simulink model "model"  (Simulink 7.3)
settings: Solver=ode45  StartTime=0.0  StopTime=2  RelTol=1e-3
values from neighbouring files (symbols this model uses):
  C_bp = 0.358    [init.m]
  C_bv = 10.71    [init.m]
  C_ep = 0.668    [init.m]
  C_ev = 20    [init.m]
  C_hp = 0.119    [init.m]
  C_hv = 3.57    [init.m]
  C_la = 19.23    [init.m]
  C_mp = 0.525    [init.m]
  C_mv = 15.71    [init.m]
  C_pa = 0.76    [init.m]
  C_pp = 5.8    [init.m]
  C_pv = 25.37    [init.m]
  C_ra = 31.25    [init.m]
  C_sa = 0.28    [init.m]
  C_sp = 2.05    [init.m]
  C_sv = 61.11    [init.m]
  D_E_max_lv = 2    [init.m]
  D_E_max_rv = 2    [init.m]
  D_R_ep = 2    [init.m]
  D_R_mp = 2    [init.m]
  D_R_sp = 2    [init.m]
  D_T_s = 2    [init.m]
  D_T_v = 0.02    [init.m]
  D_u_ev = 5    [init.m]
  D_u_mv = 5    [init.m]
  D_u_sv = 5    [init.m]
  D_v = 6    [init.m]
  E_max_lv_0 = 2.392    [init.m]
  E_max_rv_0 = 1.412    [init.m]
  f_ab_0 = 1    [init.m]
  f_abmax = 47.78    [init.m]
  f_abmin = 0    [init.m]
  f_ac_max = 17.07    [init.m]
  f_ac_min = 0    [init.m]
  f_ac_n = 3.6    [init.m]
  f_es_0 = 16.11    [init.m]
  f_es_inf = 2.1    [init.m]
  f_es_max = 60    [init.m]
  f_es_min = 0    [init.m]
  f_ev_0 = 3.2    [init.m]
  f_ev_inf = 6.3    [init.m]
  fi_sh = 0    [init.m]
  fi_sp = 0    [init.m]
  fi_v = -0.68    [init.m]
  G_ap = 23.29    [init.m]
  G_E_max_lv = 0.475    [init.m]
  G_E_max_rv = 0.282    [init.m]
  G_R_ep = 1.94    [init.m]
  G_R_mp = 2.47    [init.m]
  G_R_sp = 0.695    [init.m]
  G_T_s = -0.13    [init.m]
  G_T_v = 0.09    [init.m]
  G_u_ev = -74.21    [init.m]
  G_u_mv = -58.29    [init.m]
  G_u_sv = -265.4    [init.m]
  G_v = 0.125    [init.m]
  k_a_b = 11.76    [init.m]
  k_ac = 29.27    [init.m]
  k_e_lv = 0.014    [init.m]
  k_e_rv = 0.011    [init.m]
  k_es = 0.0675    [init.m]
  k_ev = 7.06    [init.m]
  k_r_lv = 0.000375    [init.m]
  k_r_rv = 0.0014    [init.m]
  k_sys = 0.075    [init.m]
  L_pa = 0.00018    [init.m]
  p_as_o2 = 30    [init.m]
  p_as_o2_n = 45    [init.m]
  p_n = 92    [init.m]
  P_o_lv = 1.5    [init.m]
  P_o_rv = 1.5    [init.m]
  R_bp = 6.57    [init.m]
  R_bv = 0.075    [init.m]
  R_ep_0 = 1.655    [init.m]
  R_ev = 0.04    [init.m]
  R_hp = 19.71    [init.m]
  R_hv = 0.224    [init.m]
  R_la = 0.0025    [init.m]
  R_mp_0 = 2.106    [init.m]
  R_mv = 0.05    [init.m]
  R_pa = 0.023    [init.m]
  R_pp = 0.0894    [init.m]
  R_pv = 0.0056    [init.m]
  R_ra = 0.0025    [init.m]
  R_sa = 0.06    [init.m]
  R_sp_0 = 2.49    [init.m]
  R_sv = 0.038    [init.m]
  T_0 = 0.58    [init.m]
  T_sys_0 = 0.5    [init.m]
  tau_c = 2    [init.m]
  tau_E_max_rv = 8    [init.m]
  tau_p = 2    [init.m]
  tau_pb = 2.076    [init.m]
  tau_R_ep = 6    [init.m]
  tau_R_mp = 6    [init.m]
  tau_R_sp = 6    [init.m]
  tau_T_s = 2    [init.m]
  tau_T_v = 1.5    [init.m]
  tau_u_ev = 20    [init.m]
  tau_u_mv = 20    [init.m]
  tau_u_sv = 20    [init.m]
  tau_v = 3    [init.m]
  tau_zb = 6.37    [init.m]
  V_tn = 0.583    [init.m]
  V_tot = 5300    [init.m]
  V_u_bp = 72.13    [init.m]
  V_u_bv = 294.64    [init.m]
  V_u_ep = 134.64    [init.m]
  V_u_ev_0 = 640.73    [init.m]
  V_u_hp = 24    [init.m]
  V_u_hv = 98.21    [init.m]
  V_u_la = 25    [init.m]
  V_u_lv = 16.77    [init.m]
  V_u_mp = 105.8    [init.m]
  V_u_mv_0 = 503.26    [init.m]
  V_u_pa = 0    [init.m]
  V_u_pp = 123    [init.m]
  V_u_pv = 120    [init.m]
  V_u_ra = 25    [init.m]
  V_u_rv = 40.8    [init.m]
  ... (+11 more)
(part 2 of 2)

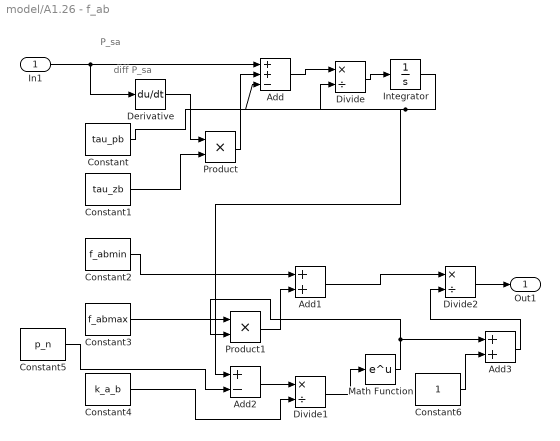
== system model/A1.26 - f_ab ==
  note: P_sa
  note: diff P_sa
  In1 : Inport  OutDataType=fixdt(1, 16)  OutScaling=2^0
  Add : Sum  Inputs=++-  OutDataType=fixdt(1, 16)  OutScaling=2^-10
  Add1 : Sum  OutDataType=fixdt(1, 16)  OutScaling=2^-10
  Add2 : Sum  Inputs=+-  OutDataType=fixdt(1, 16)  OutScaling=2^-10
  Add3 : Sum  OutDataType=fixdt(1, 16)  OutScaling=2^-10
  Constant : Constant  Value=tau_pb  OutDataType=fixdt(1, 16)  OutScaling=2^0
  Constant1 : Constant  Value=tau_zb  OutDataType=fixdt(1, 16)  OutScaling=2^0
  Constant2 : Constant  Value=f_abmin  OutDataType=fixdt(1, 16)  OutScaling=2^0
  Constant3 : Constant  Value=f_abmax  OutDataType=fixdt(1, 16)  OutScaling=2^0
  Constant4 : Constant  Value=k_a_b  OutDataType=fixdt(1, 16)  OutScaling=2^0
  Constant5 : Constant  Value=p_n  OutDataType=fixdt(1, 16)  OutScaling=2^0
  Constant6 : Constant  OutDataType=fixdt(1, 16)  OutScaling=2^0
  Derivative : Derivative
  Divide : Product  Inputs=*/  OutDataType=fixdt(1, 16)  OutScaling=2^-10
  Divide1 : Product  Inputs=*/  OutDataType=fixdt(1, 16)  OutScaling=2^-10
  Divide2 : Product  Inputs=*/  OutDataType=fixdt(1, 16)  OutScaling=2^-10
  Integrator : Integrator  InitialCondition=1
  Math Function : Math  OutDataType=fixdt(1, 16)  OutScaling=2^0  SaturateOnIntegerOverflow=on
  Product : Product  OutDataType=fixdt(1, 16)  OutScaling=2^0  RndMeth=Zero
  Product1 : Product  OutDataType=fixdt(1, 16)  OutScaling=2^0  RndMeth=Zero
  Out1 : Outport  OutDataType=fixdt(1, 16)  OutScaling=2^0
  wires:
  Constant1/1 -> Product/2
  Product/1 -> Add/2
  Integrator/1 -> Add/3, Add2/1
  Add/1 -> Divide/1
  Constant/1 -> Divide/2
  Divide/1 -> Integrator/1
  Constant2/1 -> Add1/1
  Constant3/1 -> Product1/1
  Add2/1 -> Divide1/1
  Constant5/1 -> Add2/2
  Constant4/1 -> Divide1/2
  Divide1/1 -> Math Function/1
  Math Function/1 -> Product1/2, Add3/1
  Product1/1 -> Add1/2
  Constant6/1 -> Add3/2
  Add3/1 -> Divide2/2
  Add1/1 -> Divide2/1
  Divide2/1 -> Out1/1
  Derivative/1 -> Product/1
  In1/1 -> Add/1, Derivative/1

== system model/A1.27 - f_ac ==
  Add : Sum  OutDataType=fixdt(1, 16)  OutScaling=2^-10
  Add1 : Sum  Inputs=+-  OutDataType=fixdt(1, 16)  OutScaling=2^-10
  Add2 : Sum  OutDataType=fixdt(1, 16)  OutScaling=2^-10
  Add3 : Sum  Inputs=+-  OutDataType=fixdt(1, 16)  OutScaling=2^-10
  Constant : Constant  Value=f_ac_max  OutDataType=fixdt(1, 16)  OutScaling=2^0
  Constant1 : Constant  Value=p_as_o2  OutDataType=fixdt(1, 16)  OutScaling=2^0
  Constant2 : Constant  Value=p_as_o2_n  OutDataType=fixdt(1, 16)  OutScaling=2^0
  Constant3 : Constant  Value=k_ac  OutDataType=fixdt(1, 16)  OutScaling=2^0
  Constant4 : Constant  Value=f_ac_min  OutDataType=fixdt(1, 16)  OutScaling=2^0
  Constant5 : Constant  OutDataType=fixdt(1, 16)  OutScaling=2^0
  Constant6 : Constant  Value=tau_c  OutDataType=fixdt(1, 16)  OutScaling=2^0
  Divide : Product  Inputs=*/  OutDataType=fixdt(1, 16)  OutScaling=2^-10
  Divide1 : Product  Inputs=*/  OutDataType=fixdt(1, 16)  OutScaling=2^-10
  Divide2 : Product  Inputs=*/  OutDataType=fixdt(1, 16)  OutScaling=2^-10
  Integrator : Integrator  InitialCondition=1
  Math Function : Math  OutDataType=fixdt(1, 16)  OutScaling=2^0  SaturateOnIntegerOverflow=on
  Product : Product  OutDataType=fixdt(1, 16)  OutScaling=2^0  RndMeth=Zero
  Out1 : Outport  OutDataType=fixdt(1, 16)  OutScaling=2^0
  wires:
  Constant/1 -> Add/1
  Constant1/1 -> Add1/1
  Constant2/1 -> Add1/2
  Add1/1 -> Divide/1
  Constant3/1 -> Divide/2
  Divide/1 -> Math Function/1
  Math Function/1 -> Product/2, Add2/1
  Constant4/1 -> Product/1
  Product/1 -> Add/2
  Constant5/1 -> Add2/2
  Add2/1 -> Divide1/2
  Add/1 -> Divide1/1
  Integrator/1 -> Add3/2, Out1/1
  Divide1/1 -> Add3/1
  Add3/1 -> Divide2/1
  Constant6/1 -> Divide2/2
  Divide2/1 -> Integrator/1

== system model/A1.28 - f_ap ==
  note: V_t
  In1 : Inport  OutDataType=fixdt(1, 16)  OutScaling=2^0
  Add : Sum  Inputs=-+  OutDataType=fixdt(1, 16)  OutScaling=2^-10
  Constant : Constant  Value=G_ap  OutDataType=fixdt(1, 16)  OutScaling=2^0
  Constant1 : Constant  Value=tau_p  OutDataType=fixdt(1, 16)  OutScaling=2^0
  Divide : Product  Inputs=*/  OutDataType=fixdt(1, 16)  OutScaling=2^-10
  Integrator : Integrator  InitialCondition=1
  Product : Product  OutDataType=fixdt(1, 16)  OutScaling=2^0  RndMeth=Zero
  Out1 : Outport  OutDataType=fixdt(1, 16)  OutScaling=2^0
  wires:
  Constant/1 -> Product/1
  Product/1 -> Add/2
  Integrator/1 -> Add/1, Out1/1
  Add/1 -> Divide/1
  Constant1/1 -> Divide/2
  Divide/1 -> Integrator/1
  In1/1 -> Product/2

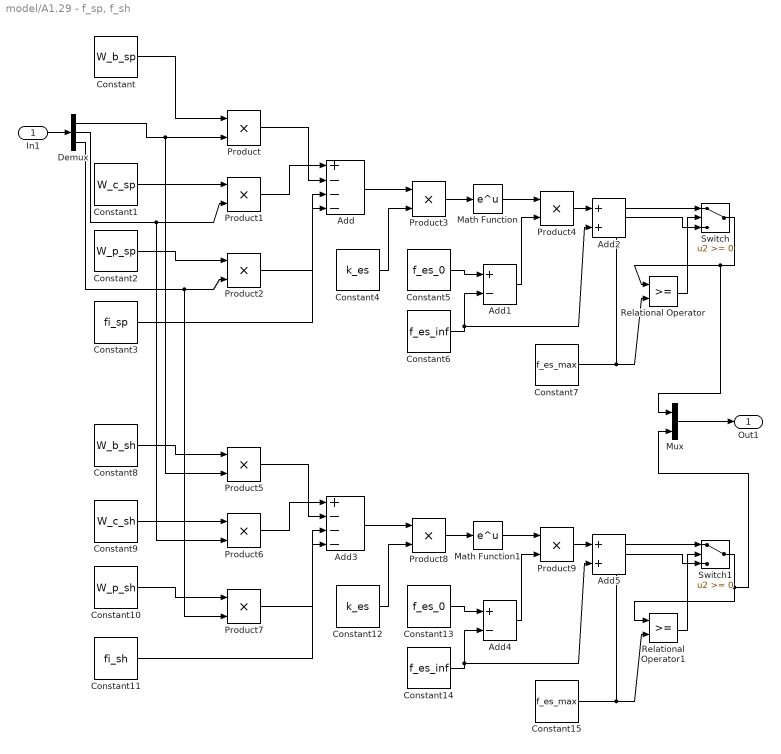
== system model/A1.29 - f_sp, f_sh ==
  In1 : Inport  OutDataType=fixdt(1, 16)  OutScaling=2^0
  Add : Sum  Inputs=+---  OutDataType=fixdt(1, 16)  OutScaling=2^-10
  Add1 : Sum  Inputs=+-  OutDataType=fixdt(1, 16)  OutScaling=2^-10
  Add2 : Sum  OutDataType=fixdt(1, 16)  OutScaling=2^-10
  Add3 : Sum  Inputs=+---  OutDataType=fixdt(1, 16)  OutScaling=2^-10
  Add4 : Sum  Inputs=+-  OutDataType=fixdt(1, 16)  OutScaling=2^-10
  Add5 : Sum  OutDataType=fixdt(1, 16)  OutScaling=2^-10
  Constant : Constant  Value=W_b_sp  OutDataType=fixdt(1, 16)  OutScaling=2^0
  Constant1 : Constant  Value=W_c_sp  OutDataType=fixdt(1, 16)  OutScaling=2^0
  Constant10 : Constant  Value=W_p_sh  OutDataType=fixdt(1, 16)  OutScaling=2^0
  Constant11 : Constant  Value=fi_sh  OutDataType=fixdt(1, 16)  OutScaling=2^0
  Constant12 : Constant  Value=k_es  OutDataType=fixdt(1, 16)  OutScaling=2^0
  Constant13 : Constant  Value=f_es_0  OutDataType=fixdt(1, 16)  OutScaling=2^0
  Constant14 : Constant  Value=f_es_inf  OutDataType=fixdt(1, 16)  OutScaling=2^0
  Constant15 : Constant  Value=f_es_max  OutDataType=fixdt(1, 16)  OutScaling=2^0
  Constant2 : Constant  Value=W_p_sp  OutDataType=fixdt(1, 16)  OutScaling=2^0
  Constant3 : Constant  Value=fi_sp  OutDataType=fixdt(1, 16)  OutScaling=2^0
  Constant4 : Constant  Value=k_es  OutDataType=fixdt(1, 16)  OutScaling=2^0
  Constant5 : Constant  Value=f_es_0  OutDataType=fixdt(1, 16)  OutScaling=2^0
  Constant6 : Constant  Value=f_es_inf  OutDataType=fixdt(1, 16)  OutScaling=2^0
  Constant7 : Constant  Value=f_es_max  OutDataType=fixdt(1, 16)  OutScaling=2^0
  Constant8 : Constant  Value=W_b_sh  OutDataType=fixdt(1, 16)  OutScaling=2^0
  Constant9 : Constant  Value=W_c_sh  OutDataType=fixdt(1, 16)  OutScaling=2^0
  Demux : Demux  Outputs=3
  Math Function : Math  OutDataType=fixdt(1, 16)  OutScaling=2^0  SaturateOnIntegerOverflow=on
  Math Function1 : Math  OutDataType=fixdt(1, 16)  OutScaling=2^0  SaturateOnIntegerOverflow=on
  Mux : Mux  Inputs=2
  Product{,1..9} (10 alike) : Product  OutDataType=fixdt(1, 16)  OutScaling=2^0  RndMeth=Zero
  Relational Operator : RelationalOperator  LogicOutDataTypeMode=boolean  LogicDataType=fixdt(0, 8)  OutDataTypeStr=boolean
  Relational Operator1 : RelationalOperator  LogicOutDataTypeMode=boolean  LogicDataType=fixdt(0, 8)  OutDataTypeStr=boolean
  Switch : Switch  OutDataType=fixdt(1, 16)  OutScaling=2^0
  Switch1 : Switch  OutDataType=fixdt(1, 16)  OutScaling=2^0
  Out1 : Outport  OutDataType=fixdt(1, 16)  OutScaling=2^0
  wires:
  In1/1 -> Demux/1
  Demux/1 -> Product/2, Product5/2
  Constant1/1 -> Product1/1
  Demux/2 -> Product1/2, Product6/2
  Constant2/1 -> Product2/1
  Demux/3 -> Product2/2, Product7/2
  Constant/1 -> Product/1
  Product1/1 -> Add/1
  Product/1 -> Add/2
  Product2/1 -> Add/3
  Constant3/1 -> Add/4
  Add/1 -> Product3/1
  Constant4/1 -> Product3/2
  Product3/1 -> Math Function/1
  Math Function/1 -> Product4/1
  Constant5/1 -> Add1/1
  Constant6/1 -> Add1/2, Add2/2
  Add1/1 -> Product4/2
  Product4/1 -> Add2/1
  Switch/1 -> Relational Operator/1, Mux/1
  Constant7/1 -> Relational Operator/2, Switch/1
  Relational Operator/1 -> Switch/2
  Add2/1 -> Switch/3
  Constant9/1 -> Product6/1
  Constant10/1 -> Product7/1
  Constant8/1 -> Product5/1
  Product6/1 -> Add3/1
  Product5/1 -> Add3/2
  Product7/1 -> Add3/3
  Constant11/1 -> Add3/4
  Add3/1 -> Product8/1
  Constant12/1 -> Product8/2
  Product8/1 -> Math Function1/1
  Math Function1/1 -> Product9/1
  Constant13/1 -> Add4/1
  Constant14/1 -> Add4/2, Add5/2
  Add4/1 -> Product9/2
  Product9/1 -> Add5/1
  Switch1/1 -> Relational Operator1/1, Mux/2
  Constant15/1 -> Relational Operator1/2, Switch1/1
  Relational Operator1/1 -> Switch1/2
  Add5/1 -> Switch1/3
  Mux/1 -> Out1/1

== system model/A1.3 - P_pp ==
  note: P pv
  note: F pa
  In1 : Inport  OutDataType=fixdt(1, 16)  OutScaling=2^0
  Constant : Constant  Value=R_pp  OutDataType=fixdt(1, 16)  OutScaling=2^0
  Constant1 : Constant  Value=C_pp  OutDataType=fixdt(1, 16)  OutScaling=2^0
  Demux : Demux  Outputs=2
  Divide : Product  Inputs=*/  OutDataType=fixdt(1, 16)  OutScaling=2^-10
  Divide1 : Product  Inputs=*/  OutDataType=fixdt(1, 16)  OutScaling=2^-10
  Integrator : Integrator  InitialCondition=1
  Subtract : Sum  Inputs=+-  OutDataType=fixdt(1, 16)  OutScaling=2^-10
  Subtract1 : Sum  Inputs=+-  OutDataType=fixdt(1, 16)  OutScaling=2^-10
  Out1 : Outport  OutDataType=fixdt(1, 16)  OutScaling=2^0
  wires:
  In1/1 -> Demux/1
  Subtract/1 -> Divide/1
  Constant/1 -> Divide/2
  Constant1/1 -> Divide1/2
  Subtract1/1 -> Divide1/1
  Divide1/1 -> Integrator/1
  Integrator/1 -> Out1/1, Subtract/1
  Divide/1 -> Subtract1/2
  Demux/1 -> Subtract/2
  Demux/2 -> Subtract1/1

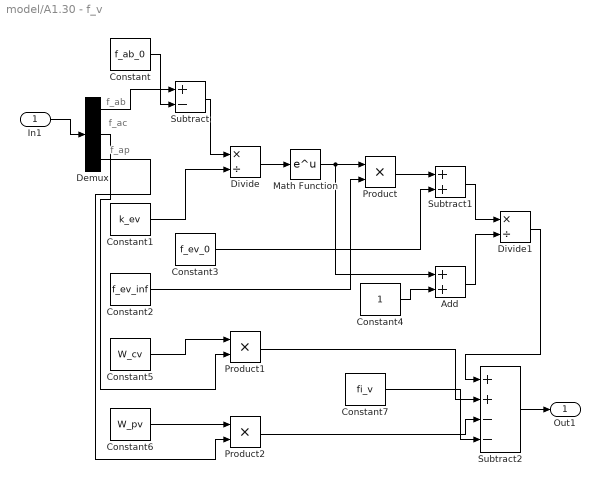
== system model/A1.30 - f_v  ==
  note: f_ab
  note: f_ac
  note: f_ap
  In1 : Inport  OutDataType=fixdt(1, 16)  OutScaling=2^0
  Add : Sum  OutDataType=fixdt(1, 16)  OutScaling=2^-10
  Constant : Constant  Value=f_ab_0  OutDataType=fixdt(1, 16)  OutScaling=2^0
  Constant1 : Constant  Value=k_ev  OutDataType=fixdt(1, 16)  OutScaling=2^0
  Constant2 : Constant  Value=f_ev_inf  OutDataType=fixdt(1, 16)  OutScaling=2^0
  Constant3 : Constant  Value=f_ev_0  OutDataType=fixdt(1, 16)  OutScaling=2^0
  Constant4 : Constant  OutDataType=fixdt(1, 16)  OutScaling=2^0
  Constant5 : Constant  Value=W_cv  OutDataType=fixdt(1, 16)  OutScaling=2^0
  Constant6 : Constant  Value=W_pv  OutDataType=fixdt(1, 16)  OutScaling=2^0
  Constant7 : Constant  Value=fi_v  OutDataType=fixdt(1, 16)  OutScaling=2^0
  Demux : Demux  Outputs=3
  Divide : Product  Inputs=*/  OutDataType=fixdt(1, 16)  OutScaling=2^-10
  Divide1 : Product  Inputs=*/  OutDataType=fixdt(1, 16)  OutScaling=2^-10
  Math Function : Math  OutDataType=fixdt(1, 16)  OutScaling=2^0  SaturateOnIntegerOverflow=on
  Product : Product  OutDataType=fixdt(1, 16)  OutScaling=2^0  RndMeth=Zero
  Product1 : Product  OutDataType=fixdt(1, 16)  OutScaling=2^0  RndMeth=Zero
  Product2 : Product  OutDataType=fixdt(1, 16)  OutScaling=2^0  RndMeth=Zero
  Subtract : Sum  Inputs=+-  OutDataType=fixdt(1, 16)  OutScaling=2^-10
  Subtract1 : Sum  OutDataType=fixdt(1, 16)  OutScaling=2^-10
  Subtract2 : Sum  Inputs=++--  OutDataType=fixdt(1, 16)  OutScaling=2^-10
  Out1 : Outport  OutDataType=fixdt(1, 16)  OutScaling=2^0
  wires:
  In1/1 -> Demux/1
  Demux/1 -> Subtract/1
  Constant/1 -> Subtract/2
  Subtract/1 -> Divide/1
  Constant1/1 -> Divide/2
  Divide/1 -> Math Function/1
  Math Function/1 -> Product/1, Add/1
  Constant2/1 -> Product/2
  Product/1 -> Subtract1/1
  Constant3/1 -> Subtract1/2
  Constant4/1 -> Add/2
  Add/1 -> Divide1/2
  Subtract1/1 -> Divide1/1
  Constant5/1 -> Product1/1
  Demux/2 -> Product1/2
  Constant6/1 -> Product2/1
  Demux/3 -> Product2/2
  Divide1/1 -> Subtract2/1
  Product1/1 -> Subtract2/2
  Product2/1 -> Subtract2/3
  Constant7/1 -> Subtract2/4
  Subtract2/1 -> Out1/1

== system model/A1.4 - P_pv ==
  note: P pp
  note: P la
  In1 : Inport  OutDataType=fixdt(1, 16)  OutScaling=2^0
  Constant : Constant  Value=R_pp  OutDataType=fixdt(1, 16)  OutScaling=2^0
  Constant1 : Constant  Value=R_pv  OutDataType=fixdt(1, 16)  OutScaling=2^0
  Constant2 : Constant  Value=C_pv  OutDataType=fixdt(1, 16)  OutScaling=2^0
  Demux : Demux  Outputs=2
  Divide : Product  Inputs=*/  OutDataType=fixdt(1, 16)  OutScaling=2^-10
  Divide1 : Product  Inputs=*/  OutDataType=fixdt(1, 16)  OutScaling=2^-10
  Divide2 : Product  Inputs=*/  OutDataType=fixdt(1, 16)  OutScaling=2^-10
  Integrator : Integrator  InitialCondition=1
  Subtract : Sum  Inputs=+-  OutDataType=fixdt(1, 16)  OutScaling=2^-10
  Subtract1 : Sum  Inputs=+-  OutDataType=fixdt(1, 16)  OutScaling=2^-10
  Subtract2 : Sum  Inputs=+-  OutDataType=fixdt(1, 16)  OutScaling=2^-10
  Out1 : Outport  OutDataType=fixdt(1, 16)  OutScaling=2^0
  wires:
  In1/1 -> Demux/1
  Demux/1 -> Subtract/1
  Demux/2 -> Subtract1/2
  Integrator/1 -> Out1/1, Subtract/2, Subtract1/1
  Subtract/1 -> Divide/1
  Constant/1 -> Divide/2
  Subtract1/1 -> Divide1/1
  Constant1/1 -> Divide1/2
  Divide/1 -> Subtract2/1
  Divide1/1 -> Subtract2/2
  Subtract2/1 -> Divide2/1
  Constant2/1 -> Divide2/2
  Divide2/1 -> Integrator/1

== system model/A1.5 - P_sa ==
  note: F o,l
  note: F sa
  In1 : Inport  OutDataType=fixdt(1, 16)  OutScaling=2^0
  Constant : Constant  Value=C_sa  OutDataType=fixdt(1, 16)  OutScaling=2^0
  Demux : Demux  Outputs=2
  Divide : Product  Inputs=*/  OutDataType=fixdt(1, 16)  OutScaling=2^-10
  Integrator : Integrator  InitialCondition=1
  Subtract : Sum  Inputs=+-  OutDataType=fixdt(1, 16)  OutScaling=2^-10
  Out1 : Outport  OutDataType=fixdt(1, 16)  OutScaling=2^0
  wires:
  In1/1 -> Demux/1
  Demux/1 -> Subtract/1
  Demux/2 -> Subtract/2
  Subtract/1 -> Divide/1
  Constant/1 -> Divide/2
  Divide/1 -> Integrator/1
  Integrator/1 -> Out1/1

== system model/A1.6 - F_sa ==
  note: P sa
  note: P sp
  note: F sa
  In1 : Inport  OutDataType=fixdt(1, 16)  OutScaling=2^0
  Constant : Constant  Value=R_sa  OutDataType=fixdt(1, 16)  OutScaling=2^0
  Demux : Demux  Outputs=2
  Integrator : Integrator  InitialCondition=1
  Product : Product  OutDataType=fixdt(1, 16)  OutScaling=2^0  RndMeth=Zero
  Subtract : Sum  Inputs=+-  OutDataType=fixdt(1, 16)  OutScaling=2^-10
  Subtract1 : Sum  Inputs=+-  OutDataType=fixdt(1, 16)  OutScaling=2^-10
  Out1 : Outport  OutDataType=fixdt(1, 16)  OutScaling=2^0
  wires:
  In1/1 -> Demux/1
  Demux/1 -> Subtract/1
  Demux/2 -> Subtract/2
  Constant/1 -> Product/1
  Subtract/1 -> Subtract1/1
  Product/1 -> Subtract1/2
  Subtract1/1 -> Integrator/1
  Integrator/1 -> Out1/1, Product/2

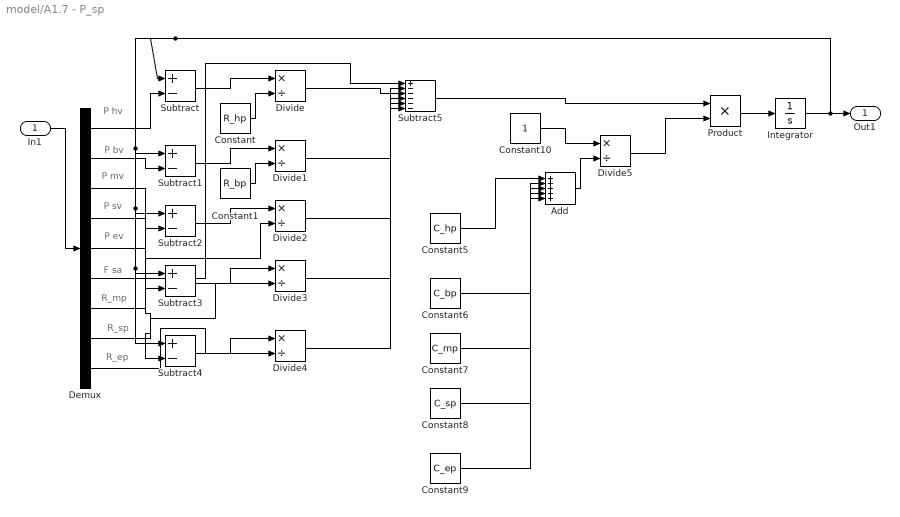
== system model/A1.7 - P_sp ==
  note: P hv
  note: P bv
  note: P mv
  note: P sv
  note: P ev
  note: F sa
  note: R_mp
  note: R_sp
  note: R_ep
  In1 : Inport  OutDataType=fixdt(1, 16)  OutScaling=2^0
  Add : Sum  Inputs=+++++  OutDataType=fixdt(1, 16)  OutScaling=2^-10
  Constant : Constant  Value=R_hp  OutDataType=fixdt(1, 16)  OutScaling=2^0
  Constant1 : Constant  Value=R_bp  OutDataType=fixdt(1, 16)  OutScaling=2^0
  Constant10 : Constant  OutDataType=fixdt(1, 16)  OutScaling=2^0
  Constant5 : Constant  Value=C_hp  OutDataType=fixdt(1, 16)  OutScaling=2^0
  Constant6 : Constant  Value=C_bp  OutDataType=fixdt(1, 16)  OutScaling=2^0
  Constant7 : Constant  Value=C_mp  OutDataType=fixdt(1, 16)  OutScaling=2^0
  Constant8 : Constant  Value=C_sp  OutDataType=fixdt(1, 16)  OutScaling=2^0
  Constant9 : Constant  Value=C_ep  OutDataType=fixdt(1, 16)  OutScaling=2^0
  Demux : Demux  Outputs=9
  Divide{,1..5} (6 alike) : Product  Inputs=*/  OutDataType=fixdt(1, 16)  OutScaling=2^-10
  Integrator : Integrator  InitialCondition=1
  Product : Product  OutDataType=fixdt(1, 16)  OutScaling=2^0  RndMeth=Zero
  Subtract{,1..4} (5 alike) : Sum  Inputs=+-  OutDataType=fixdt(1, 16)  OutScaling=2^-10
  Subtract5 : Sum  Inputs=+-----  OutDataType=fixdt(1, 16)  OutScaling=2^-10
  Out1 : Outport  OutDataType=fixdt(1, 16)  OutScaling=2^0
  wires:
  In1/1 -> Demux/1
  Constant/1 -> Divide/2
  Subtract/1 -> Divide/1
  Constant1/1 -> Divide1/2
  Subtract1/1 -> Divide1/1
  Subtract2/1 -> Divide2/1
  Subtract3/1 -> Divide3/1
  Subtract4/1 -> Divide4/1
  Divide/1 -> Subtract5/2
  Divide1/1 -> Subtract5/3
  Divide2/1 -> Subtract5/4
  Divide3/1 -> Subtract5/5
  Divide4/1 -> Subtract5/6
  Constant5/1 -> Add/1
  Constant6/1 -> Add/2
  Constant7/1 -> Add/3
  Constant8/1 -> Add/4
  Constant9/1 -> Add/5
  Constant10/1 -> Divide5/1
  Add/1 -> Divide5/2
  Subtract5/1 -> Product/1
  Divide5/1 -> Product/2
  Product/1 -> Integrator/1
  Integrator/1 -> Out1/1, Subtract/1, Subtract1/1, Subtract2/1, Subtract3/1, Subtract4/1
  Demux/1 -> Subtract/2
  Demux/2 -> Subtract1/2
  Demux/3 -> Subtract2/2
  Demux/4 -> Subtract3/2
  Demux/5 -> Subtract4/2
  Demux/6 -> Subtract5/1
  Demux/7 -> Divide2/2
  Demux/8 -> Divide3/2
  Demux/9 -> Divide4/2

== system model/A1.8 - P_hv ==
  note: P sp
  note: P ra
  In1 : Inport  OutDataType=fixdt(1, 16)  OutScaling=2^0
  Constant : Constant  Value=R_hp  OutDataType=fixdt(1, 16)  OutScaling=2^0
  Constant1 : Constant  Value=R_hv  OutDataType=fixdt(1, 16)  OutScaling=2^0
  Constant2 : Constant  Value=C_hv  OutDataType=fixdt(1, 16)  OutScaling=2^0
  Demux : Demux  Outputs=2
  Divide : Product  Inputs=*/  OutDataType=fixdt(1, 16)  OutScaling=2^-10
  Divide1 : Product  Inputs=*/  OutDataType=fixdt(1, 16)  OutScaling=2^-10
  Divide2 : Product  Inputs=*/  OutDataType=fixdt(1, 16)  OutScaling=2^-10
  Integrator : Integrator  InitialCondition=1
  Subtract : Sum  Inputs=+-  OutDataType=fixdt(1, 16)  OutScaling=2^-10
  Subtract1 : Sum  Inputs=+-  OutDataType=fixdt(1, 16)  OutScaling=2^-10
  Subtract2 : Sum  Inputs=+-  OutDataType=fixdt(1, 16)  OutScaling=2^-10
  Out1 : Outport  OutDataType=fixdt(1, 16)  OutScaling=2^0
  wires:
  In1/1 -> Demux/1
  Demux/1 -> Subtract/1
  Subtract/1 -> Divide/1
  Constant1/1 -> Divide1/2
  Constant/1 -> Divide/2
  Subtract1/1 -> Divide1/1
  Divide/1 -> Subtract2/1
  Divide1/1 -> Subtract2/2
  Subtract2/1 -> Divide2/1
  Constant2/1 -> Divide2/2
  Divide2/1 -> Integrator/1
  Integrator/1 -> Out1/1, Subtract/2, Subtract1/1
  Demux/2 -> Subtract1/2

== system model/A1.9 - P_bv ==
  note: P sp
  note: P ra
  In1 : Inport  OutDataType=fixdt(1, 16)  OutScaling=2^0
  Constant : Constant  Value=R_bp  OutDataType=fixdt(1, 16)  OutScaling=2^0
  Constant1 : Constant  Value=R_bv  OutDataType=fixdt(1, 16)  OutScaling=2^0
  Constant2 : Constant  Value=C_bv  OutDataType=fixdt(1, 16)  OutScaling=2^0
  Demux : Demux  Outputs=2
  Divide : Product  Inputs=*/  OutDataType=fixdt(1, 16)  OutScaling=2^-10
  Divide1 : Product  Inputs=*/  OutDataType=fixdt(1, 16)  OutScaling=2^-10
  Divide2 : Product  Inputs=*/  OutDataType=fixdt(1, 16)  OutScaling=2^-10
  Integrator : Integrator  InitialCondition=1
  Subtract : Sum  Inputs=+-  OutDataType=fixdt(1, 16)  OutScaling=2^-10
  Subtract1 : Sum  Inputs=+-  OutDataType=fixdt(1, 16)  OutScaling=2^-10
  Subtract2 : Sum  Inputs=+-  OutDataType=fixdt(1, 16)  OutScaling=2^-10
  Out1 : Outport  OutDataType=fixdt(1, 16)  OutScaling=2^0
  wires:
  In1/1 -> Demux/1
  Demux/1 -> Subtract/1
  Subtract/1 -> Divide/1
  Constant1/1 -> Divide1/2
  Constant/1 -> Divide/2
  Subtract1/1 -> Divide1/1
  Divide/1 -> Subtract2/1
  Divide1/1 -> Subtract2/2
  Subtract2/1 -> Divide2/1
  Constant2/1 -> Divide2/2
  Divide2/1 -> Integrator/1
  Integrator/1 -> Out1/1, Subtract/2, Subtract1/1
  Demux/2 -> Subtract1/2
